simulink model "untitled"  (R2024a)
settings: Solver=FixedStepAuto  StartTime=0.0  StopTime=30  FixedStep=0.01  MaxStep=0  MinStep=0.0001  RelTol=1e-3
libraries: simulink x7
settings Model: Creator=ventus  LastModifiedBy=ventus

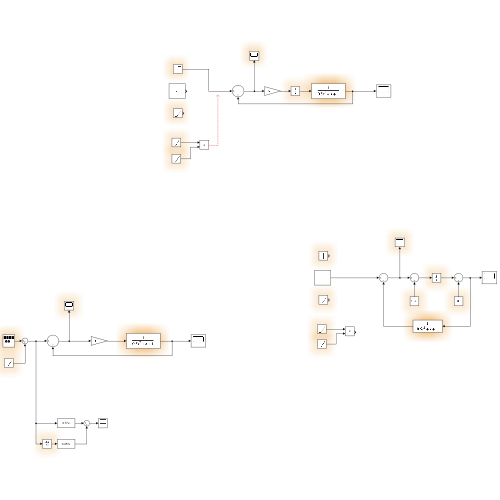
[thumbnail: Simulink's stored preview of the top-level diagram]
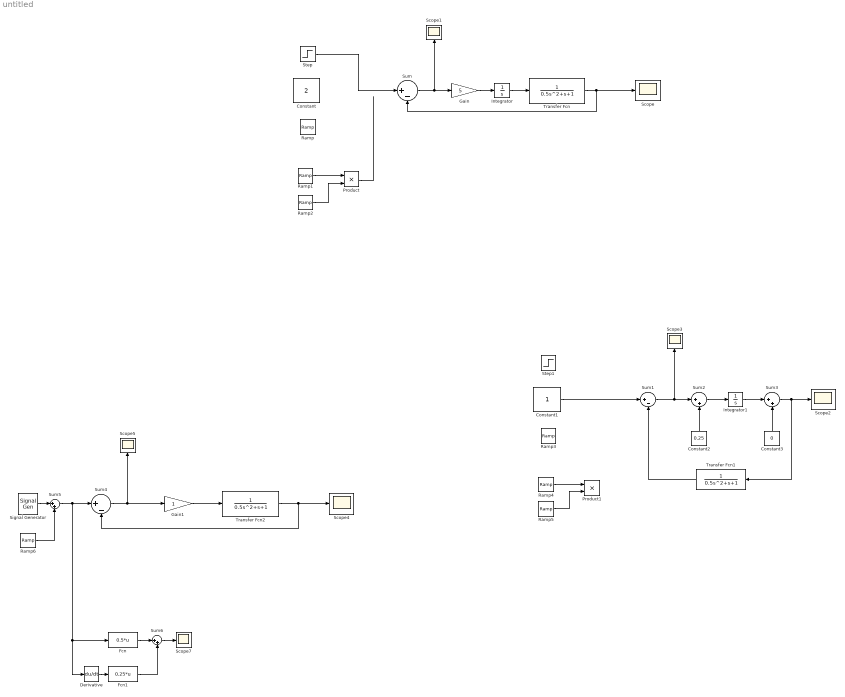
== system untitled ==
  Constant : Constant  Value=2
  Constant1 : Constant
  Constant2 : Constant  Value=0.25
  Constant3 : Constant  Value=0
  Derivative : Derivative
  Fcn : Fcn  Expr=0.5*u
  Fcn1 : Fcn  Expr=0.25*u
  Gain : Gain  Gain=5
  Gain1 : Gain
  Integrator : Integrator
  Integrator1 : Integrator
  Product : Product
  Product1 : Product
  Ramp : simulink/Sources/Ramp  slope=2  start=0  InitialOutput=0
  Ramp1 : simulink/Sources/Ramp  slope=0.45  start=0  InitialOutput=0
  Ramp2 : simulink/Sources/Ramp  slope=1  start=0  InitialOutput=0
  Ramp3 : simulink/Sources/Ramp  slope=2  start=0  InitialOutput=0
  Ramp4 : simulink/Sources/Ramp  slope=0.45  start=0  InitialOutput=0
  Ramp5 : simulink/Sources/Ramp  slope=1  start=0  InitialOutput=0
  Ramp6 : simulink/Sources/Ramp  slope=0.3  start=0  InitialOutput=0
  Scope{,1..5,7} (7 alike) : Scope
  Signal Generator : SignalGenerator  Amplitude=2  Frequency=0.8  Units=rad/sec
  Step : Step  SampleTime=0
  Step1 : Step  SampleTime=0
  Sum : Sum  Inputs=|+-
  Sum1 : Sum  Inputs=|+-
  Sum{2..3,5..6} (4 alike) : Sum  Inputs=|++
  Sum4 : Sum  Inputs=|+-
  Transfer Fcn : TransferFcn  Denominator=[0.5 1 1]
  Transfer Fcn1 : TransferFcn  Denominator=[0.5 1 1]
  Transfer Fcn2 : TransferFcn  Denominator=[0.5 1 1]
  wires:
  Sum/1 -> Gain/1, Scope1/1
  Transfer Fcn/1 -> Sum/2, Scope/1
  Gain/1 -> Integrator/1
  Integrator/1 -> Transfer Fcn/1
  Ramp1/1 -> Product/1
  Ramp2/1 -> Product/2
  Product/1 -> ?
  Ramp5/1 -> Product1/2
  Ramp4/1 -> Product1/1
  Sum1/1 -> Scope3/1, Sum2/1
  Sum2/1 -> Integrator1/1
  Sum3/1 -> Transfer Fcn1/1, Scope2/1
  Integrator1/1 -> Sum3/1
  Transfer Fcn1/1 -> Sum1/2
  Constant2/1 -> Sum2/2
  Constant3/1 -> Sum3/2
  Constant1/1 -> Sum1/1
  Gain1/1 -> Transfer Fcn2/1
  Transfer Fcn2/1 -> Sum4/2, Scope4/1
  Sum4/1 -> Gain1/1, Scope5/1
  Signal Generator/1 -> Sum5/1
  Ramp6/1 -> Sum5/2
  Sum5/1 -> Derivative/1, Fcn/1, Sum4/1
  Derivative/1 -> Fcn1/1
  Fcn/1 -> Sum6/1
  Fcn1/1 -> Sum6/2
  Sum6/1 -> Scope7/1
  Step/1 -> Sum/1
